simulink model "GMPP2"  (Simulink 8.7)
settings: Solver=ode15s  StartTime=0.0  StopTime=0.3  RelTol=1e-3
libraries: powerlib x29, simulink x13, neural x6
(part 1 of 2)
settings Model: Creator=Loubna  LastModifiedBy=dell
settings DebuggingCC: UnderspecifiedInitializationDetection=Simplified  MergeDetectMultiDrivingBlocksExec=error  SolverPrmCheckMsg=warning
settings ConfigComp: CovSFcnEnable=off

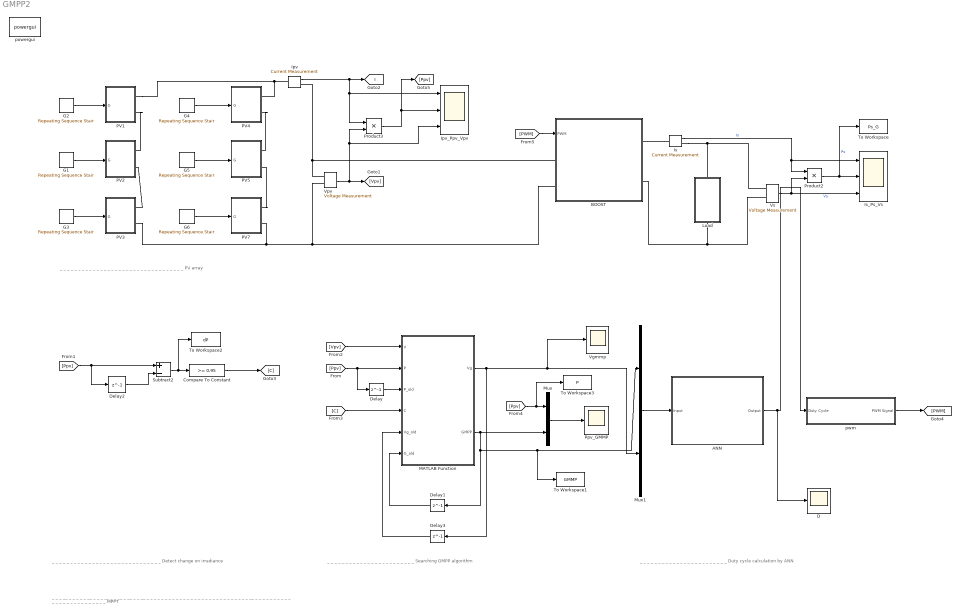
== system GMPP2 ==
  note: _ _ _ _ _ _ _ _ _ _ _ _ _ _ _ _ _ _ _ _ _ _ _ _ _ _ _ _ _ _
      | Detect change on irradiance
  note: _ _ _ _ _ _ _ _ _ _ _ _ _ _ _ _ _ _ _ _ _ _ _ _ _ _ _ _ _ _ _ _ _ _
      | PV array
  note: _ _ _ _ _ _ _ _ _ _ _ _ _ _ _ _ _ _ _ _ _ _ _ _
      | Searching GMPP algorithm
  note: _ _ _ _ _ _ _ _ _ _ _ _ _ _ _ _ _ _ _ _ _ _ _ _
      | Duty cycle calculation by ANN
  note: _ _ _ __ _ _ _ _ _ __ _ _ _ __ _ _ __ _ __ _ _ __ _ _ _ _ _ _ _ _ _ _ _ _ _ _ _ _ _ _ _ _ _ _ _ _ _ _ _ _ __ _ _ _ _ _ _ _ _ _ _ _ _ _ _ _ _ _ _ _ _ _ _ _ _ _
      | MPPT
  ANN : Subsystem
      mask help: Function Fitting Neural Network
      mask Display: e = 0.06;c1 = [120 150 230]/255;c2 = ([120 150 230]+0)/383;c3 = ([120 150 230]+128)/383;patch([0 1 1 0],[0 0 1 1],c1);patch([0 1 1 1-e 1-e 0+e],[0 0 1 1-e 0+e 0+e],c2);patch([0 0 1 1-e 0+e 0+e],[0 1 1 1-e 1-e 0+e],c3);plot([0 1 1 0 0],[0 0 1 1 0]);fprintf('NNET');port_label('input',1,' Input');port_label('output',1,'Output ');
  BOOST : Subsystem
  Compare To Constant : simulink/Logic and Bit Operations/Compare To Constant  relop=>=  const=0.95  OutDataTypeStr=boolean
  D : Scope
  Delay : Delay  DelayLength=1  InitialCondition=0  SampleTime=1e-7
  Delay1 : Delay  DelayLength=1  InitialCondition=0  SampleTime=1e-6
  Delay2 : Delay  DelayLength=1  InitialCondition=0  SampleTime=1e-7
  Delay3 : Delay  DelayLength=1  InitialCondition=0  SampleTime=1e-6
  G1 : simulink/Sources/Repeating Sequence Stair  OutValues=[520 800 560]  tsamp=0.1  OutMin=[]  OutMax=[]  OutDataTypeStr=double  OutputDataTypeScalingMode=double  OutDataType=fixdt(0,8)  ConRadixGroup=Best Precision: Vector-wise  OutScaling=2^-12
  G2 : simulink/Sources/Repeating Sequence Stair  OutValues=[400 550 720]  tsamp=0.1  OutMin=[]  OutMax=[]  OutDataTypeStr=double  OutputDataTypeScalingMode=double  OutDataType=fixdt(0,8)  ConRadixGroup=Best Precision: Vector-wise  OutScaling=2^-12
  G3 : simulink/Sources/Repeating Sequence Stair  OutValues=[700 800 600]  tsamp=0.1  OutMin=[]  OutMax=[]  OutDataTypeStr=double  OutputDataTypeScalingMode=double  OutDataType=fixdt(0,8)  ConRadixGroup=Best Precision: Vector-wise  OutScaling=2^-12
  G4 : simulink/Sources/Repeating Sequence Stair  OutValues=[400 550 560]  tsamp=0.1  OutMin=[]  OutMax=[]  OutDataTypeStr=double  OutputDataTypeScalingMode=double  OutDataType=fixdt(0,8)  ConRadixGroup=Best Precision: Vector-wise  OutScaling=2^-12
  G5 : simulink/Sources/Repeating Sequence Stair  OutValues=[520 800 600]  tsamp=0.1  OutMin=[]  OutMax=[]  OutDataTypeStr=double  OutputDataTypeScalingMode=double  OutDataType=fixdt(0,8)  ConRadixGroup=Best Precision: Vector-wise  OutScaling=2^-12
  G6 : simulink/Sources/Repeating Sequence Stair  OutValues=[700 800 400]  tsamp=0.1  OutMin=[]  OutMax=[]  OutDataTypeStr=double  OutputDataTypeScalingMode=double  OutDataType=fixdt(0,8)  ConRadixGroup=Best Precision: Vector-wise  OutScaling=2^-12
  Ipv : powerlib/Measurements/Current Measurement  PhasorSimulation=off  OutputType=Complex  PSBequivalent=0
  Ipv_Ppv_Vpv : Scope  NumInputPorts=3
  Is : powerlib/Measurements/Current Measurement  PhasorSimulation=off  OutputType=Complex  PSBequivalent=0
  Is_Ps_Vs : Scope  NumInputPorts=3
  Load : Subsystem
  MATLAB Function : MATLAB Function  TreatAsAtomicUnit=on
  Mux : Mux  Inputs=2
  Mux1 : Mux  Inputs=2
  PV1 : Subsystem
  PV2 : Subsystem
  PV3 : Subsystem
  PV4 : Subsystem
  PV5 : Subsystem
  PV7 : Subsystem
  Ppv_GMMP : Scope
  Product2 : Product
  Product3 : Product
  Subtract2 : Sum  Inputs=+-
  To Workspace : ToWorkspace  VariableName=Ps_G  SaveFormat=Timeseries  SampleTime=-1
  To Workspace1 : ToWorkspace  VariableName=GMMP  SaveFormat=Timeseries  SampleTime=-1
  To Workspace2 : ToWorkspace  VariableName=dP  SaveFormat=Timeseries  SampleTime=-1
  To Workspace3 : ToWorkspace  VariableName=P  SaveFormat=Timeseries  SampleTime=-1
  Vgmmp : Scope
  Vpv : powerlib/Measurements/Voltage Measurement  Tag=PoWeRsYsTeMmEaSuReMeNt  PhasorSimulation=off  OutputType=Magnitude  PSBequivalent=0
  Vs : powerlib/Measurements/Voltage Measurement  Tag=PoWeRsYsTeMmEaSuReMeNt  PhasorSimulation=off  OutputType=Magnitude  PSBequivalent=0
  powergui : powerlib/powergui  Priority=1  SimulationMode=Discrete  SolverType=Tustin  SampleTime=1e-6  frequency=60  SPID=off  DisableSnubberDevices=off  DisableRonSwitches=off  DisableVfSwitches=off  SwTol=0  DisplayEquations=off  Interpol=off  ExternalGateDelay=off  methode=off  Ts=0  FunctionMessages=off  echomessages=off  HookPort=off  EnableUseOfTLC=off  x0status=blocks  frequencyindice=0  Pbase=100e6  ErrMax=1e-4  Iterations=50  UnitsV=kV  UnitsW=MW  buscounter=0  RestoreLinks=warning  ResistiveCurrentMeasurement=off  Frange=[0:2:500]  Ylog=off  Xlog=on  ShowGrid=off  save=off  variable=ZData  structure=0  ZoomFFT=off  StartTime=0.0  cycles=1  DisplayStyle=1  fundamental=60  FreqAxis=off  MaxFrequency=1000  frequencyindicesteady=1  RmsSteady=1  display=off
  pwm : Subsystem  mask(PWM Generator for non bridge applications){fs=20000, A=1}
      mask prompts: fs "Frequency"; A "Amplitude"
      mask help:
      | By default it outputs a 1 unit square wave at 1 hz
      | You can set the duty cycle or use an external line to ajust it on the fly.
  tag scope: I=global
  wires:
  Ipv/1 -> Product3/1, Ipv_Ppv_Vpv/1, [I]
  Vpv/1 -> Product3/2, Ipv_Ppv_Vpv/3, [Vpv]
  [Ppv] -> Subtract2/1, Delay2/1
  Delay2/1 -> Subtract2/2
  Subtract2/1 -> To Workspace2/1, Compare To Constant/1
  Delay/1 -> MATLAB Function/3(P_old)
  Delay1/1 -> MATLAB Function/6(G_old)
  Mux/1 -> Ppv_GMMP/1
  [Ppv] -> Delay/1, MATLAB Function/2(P)
  [Vpv] -> MATLAB Function/1(V)
  Mux1/1 -> ANN/1(Input)
  ANN/1(Output) -> pwm/1(Duty Cycle), D/1
  Product2/1 -> To Workspace/1, Is_Ps_Vs/2  "Ps"
  Vs/1 -> Is_Ps_Vs/3, Product2/2  "Vs"
  Is/1 -> Is_Ps_Vs/1, Product2/1  "Is"
  Product3/1 -> [Ppv], Ipv_Ppv_Vpv/2
  Compare To Constant/1 -> [C]
  MATLAB Function/2(GMPP) -> Delay1/1, To Workspace1/1, Mux1/1, Mux/2
  MATLAB Function/1(Vg) -> Delay3/1, Mux1/2, Vgmmp/1
  Delay3/1 -> MATLAB Function/5(Vg_old)
  [Ppv] -> To Workspace3/1, Mux/1
  pwm/1(PWM Signal) -> [PWM]
  [PWM] -> BOOST/1(PWM)
  [C] -> MATLAB Function/4(C)
  G2/1 -> PV1/1(G)
  G3/1 -> PV3/1(G)
  G4/1 -> PV4/1(G)
  G5/1 -> PV5/1(G)
  G6/1 -> PV7/1(G)
  G1/1 -> PV2/1(G)
  connections:
  Vpv/LConn1 -- BOOST/LConn1 -- Ipv/RConn1
  Ipv/LConn1 -- PV4/RConn1 -- PV1/RConn1
  BOOST/LConn2 -- PV3/RConn2 -- PV7/RConn2 -- Vpv/LConn2
  PV1/RConn2 -- PV2/RConn1
  PV4/RConn2 -- PV5/RConn1
  PV7/RConn1 -- PV5/RConn2
  PV3/RConn1 -- PV2/RConn2
  Vs/LConn1 -- Is/RConn1 -- Load/LConn1
  Is/LConn1 -- BOOST/RConn1
  Vs/LConn2 -- BOOST/RConn2 -- Load/RConn1

== system GMPP2/ANN ==
  Input : Inport  PortDimensions=2
      mask Display: e = 0.06;c1 = [120 230 180]/255;c2 = ([120 230 180]+0)/(256+128);c3 = ([120 230 180]+128)/(256+128);patch([0 1 1 0],[0 0 1 1],c1);patch([0 1 1 1-e 1-e 0+e],[0 0 1 1-e 0+e 0+e],c2);patch([0 0 1 1-e 0+e 0+e],[0 1 1 1-e 1-e 0+e],c3);plot([0 1 1 0 0],[0 0 1 1 0]);
  Layer 1 : Subsystem
      mask Display: e = 0.06;c1 = [120 150 230]/255;c2 = ([120 150 230]+0)/383;c3 = ([120 150 230]+128)/383;patch([0 1 1 0],[0 0 1 1],c1);patch([0 1 1 1-e 1-e 0+e],[0 0 1 1-e 0+e 0+e],c2);patch([0 0 1 1-e 0+e 0+e],[0 1 1 1-e 1-e 0+e],c3);plot([0 1 1 0 0],[0 0 1 1 0]);
  Layer 2 : Subsystem
      mask Display: e = 0.06;c1 = [120 150 230]/255;c2 = ([120 150 230]+0)/383;c3 = ([120 150 230]+128)/383;patch([0 1 1 0],[0 0 1 1],c1);patch([0 1 1 1-e 1-e 0+e],[0 0 1 1-e 0+e 0+e],c2);patch([0 0 1 1-e 0+e 0+e],[0 1 1 1-e 1-e 0+e],c3);plot([0 1 1 0 0],[0 0 1 1 0]);
  Process Input 1 : Subsystem
      mask Display: e = 0.06;c1 = [120 150 230]/255;c2 = ([120 150 230]+0)/383;c3 = ([120 150 230]+128)/383;patch([0 1 1 0],[0 0 1 1],c1);patch([0 1 1 1-e 1-e 0+e],[0 0 1 1-e 0+e 0+e],c2);patch([0 0 1 1-e 0+e 0+e],[0 1 1 1-e 1-e 0+e],c3);plot([0 1 1 0 0],[0 0 1 1 0]);
  Process Output 1 : Subsystem
      mask Display: e = 0.06;c1 = [120 150 230]/255;c2 = ([120 150 230]+0)/383;c3 = ([120 150 230]+128)/383;patch([0 1 1 0],[0 0 1 1],c1);patch([0 1 1 1-e 1-e 0+e],[0 0 1 1-e 0+e 0+e],c2);patch([0 0 1 1-e 0+e 0+e],[0 1 1 1-e 1-e 0+e],c3);plot([0 1 1 0 0],[0 0 1 1 0]);
  Output : Outport  InitialOutput=0
      mask Display: e = 0.06;c1 = [120 230 180]/255;c2 = ([120 230 180]+0)/(256+128);c3 = ([120 230 180]+128)/(256+128);patch([0 1 1 0],[0 0 1 1],c1);patch([0 1 1 1-e 1-e 0+e],[0 0 1 1-e 0+e 0+e],c2);patch([0 0 1 1-e 0+e 0+e],[0 1 1 1-e 1-e 0+e],c3);plot([0 1 1 0 0],[0 0 1 1 0]);
  wires:
  Input/1 -> Process Input 1/1(x)
  Process Output 1/1(y) -> Output/1
  Process Input 1/1(p) -> Layer 1/1("p{1}")
  Layer 1/1("a{1}") -> [feedback1]
  [feedback1] -> Layer 2/1("a{1} ")
  Layer 2/1("a{2}") -> Process Output 1/1(a)

== system GMPP2/BOOST ==
  PWM : Inport
  Ce : powerlib/Elements/Series RLC Branch  LConnTagsString=__new0  RConnTagsString=__new0  BranchType=C  Resistance=0.01  Inductance=1.0  SetiL0=off  InitialCurrent=0  Capacitance=10e-6  Setx0=off  InitialVoltage=0  Measurements=None
  Cs : powerlib/Elements/Series RLC Branch  LConnTagsString=__new0  RConnTagsString=__new0  BranchType=C  Resistance=0.01  Inductance=1.0  SetiL0=off  InitialCurrent=0  Capacitance=200e-6  Setx0=off  InitialVoltage=0  Measurements=None
  Diode : powerlib/Power Electronics/Diode  Ron=0.001  Lon=0  Vf=0.8  IC=0  UseSnubber=off  Rs=500  Cs=250e-9  Measurements=off
  Ideal Switch : powerlib/Power Electronics/Ideal Switch  Ron=0.001  Lon=0  IC=0  Rs=1e5  Cs=inf  Measurements=off
  L : powerlib/Elements/Series RLC Branch  LConnTagsString=__new0  RConnTagsString=__new0  BranchType=L  Resistance=0.01  Inductance=10e-3  SetiL0=on  InitialCurrent=0  Capacitance=25e-6  Setx0=off  InitialVoltage=0  Measurements=None
  Vpv+ : PMIOPort  Port=1  Side=Left
  Vs+ : PMIOPort  Port=2  Side=Right
  Vpv- : PMIOPort  Port=3  Side=Left
  Vs- : PMIOPort  Port=4  Side=Right
  wires:
  PWM/1 -> Ideal Switch/1
  connections:
  Diode/LConn1 -- L/LConn1 -- Ideal Switch/LConn1
  Cs/LConn1 -- Vs+/RConn1 -- Diode/RConn1
  Vpv-/RConn1 -- Cs/RConn1 -- Vs-/RConn1 -- Ideal Switch/RConn1 -- Ce/RConn1
  L/RConn1 -- Ce/LConn1 -- Vpv+/RConn1

== system GMPP2/Load ==
  R : powerlib/Elements/Series RLC Branch  LConnTagsString=__new0  RConnTagsString=__new0  BranchType=R  Resistance=15  Inductance=1.0  SetiL0=off  InitialCurrent=0  Capacitance=80e-6  Setx0=off  InitialVoltage=0  Measurements=None
  Vs+ : PMIOPort  Port=1  Side=Left
  Vs- : PMIOPort  Port=2  Side=Right
  connections:
  R/RConn1 -- Vs-/RConn1
  Vs+/RConn1 -- R/LConn1

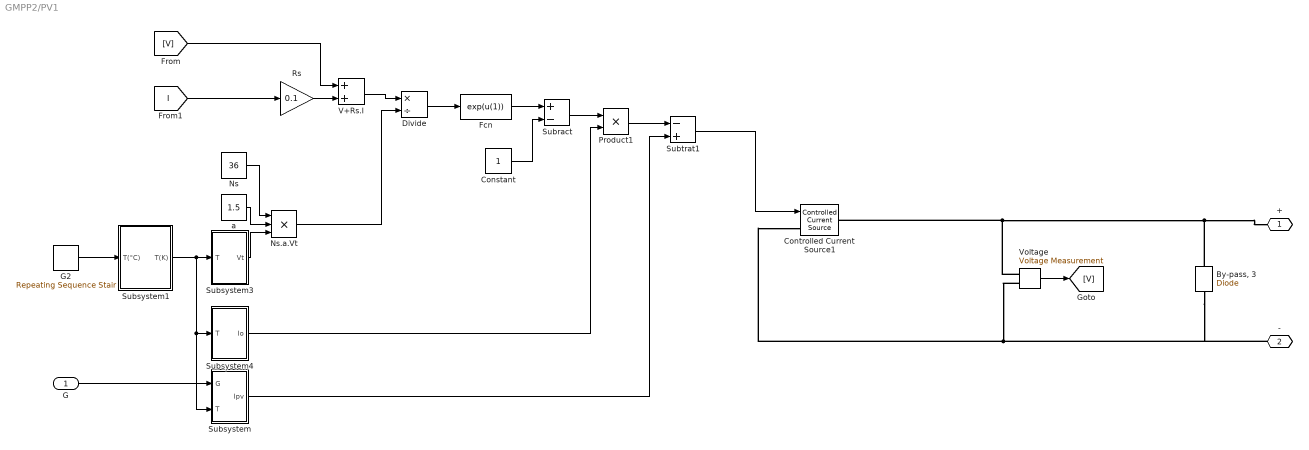
== system GMPP2/PV1 ==
  G : Inport
  "By-pass, 3" : powerlib/Power Electronics/Diode  Ron=0.01  Lon=10e-3  Vf=0.6  IC=0  UseSnubber=off  Rs=0  Cs=250e-9  Measurements=off
  Constant : Constant
  Controlled Current Source1 : powerlib/Electrical Sources/Controlled Current Source  Initialize=on  Source_Type=AC  Amplitude=0  Phase=0  Frequency=0  Measurements=None
  Divide : Product  Inputs=*/
  Fcn : Fcn  Expr=exp(u(1))
  G2 : simulink/Sources/Repeating Sequence Stair  OutValues=[25]  tsamp=0.1  OutMin=[]  OutMax=[]  OutDataTypeStr=double  OutputDataTypeScalingMode=double  OutDataType=fixdt(0,8)  ConRadixGroup=Best Precision: Vector-wise  OutScaling=2^-12
  Ns : Constant  Value=36
  Ns.a.Vt : Product  Inputs=3  RndMeth=Zero
  Product1 : Product  RndMeth=Zero
  Rs : Gain  Gain=0.1
  Subract : Sum  Inputs=+-
  Subsystem : Subsystem
  Subsystem1 : Subsystem
  Subsystem3 : Subsystem
  Subsystem4 : Subsystem
  Subtrat1 : Sum  Inputs=-+
  V+Rs.I : Sum
  "Voltage " : powerlib/Measurements/Voltage Measurement  PhasorSimulation=off  OutputType=Complex  PSBequivalent=0
  a : Constant  Value=1.5
  + : PMIOPort  Port=1  Side=Right
  - : PMIOPort  Port=2  Side=Right
  wires:
  V+Rs.I/1 -> Divide/1
  Divide/1 -> Fcn/1
  Fcn/1 -> Subract/1
  Constant/1 -> Subract/2
  Subract/1 -> Product1/1
  Subsystem4/1(Io) -> Product1/2
  Product1/1 -> Subtrat1/1
  Subsystem1/1(T(K)) -> Subsystem3/1(T), Subsystem4/1(T), Subsystem/2(T)
  G/1 -> Subsystem/1(G)
  Subtrat1/1 -> Controlled Current Source1/1
  G2/1 -> Subsystem1/1(T(°C))
  Ns/1 -> Ns.a.Vt/1
  a/1 -> Ns.a.Vt/2
  Subsystem3/1(Vt) -> Ns.a.Vt/3
  Subsystem/1(Ipv) -> Subtrat1/2
  "Voltage "/1 -> [V]
  Rs/1 -> V+Rs.I/2
  Ns.a.Vt/1 -> Divide/2
  [I] -> Rs/1
  [V] -> V+Rs.I/1
  connections:
  "Voltage "/LConn2 -- -/RConn1 -- "By-pass, 3"/LConn1 -- Controlled Current Source1/LConn1
  "Voltage "/LConn1 -- Controlled Current Source1/RConn1 -- "By-pass, 3"/RConn1 -- +/RConn1

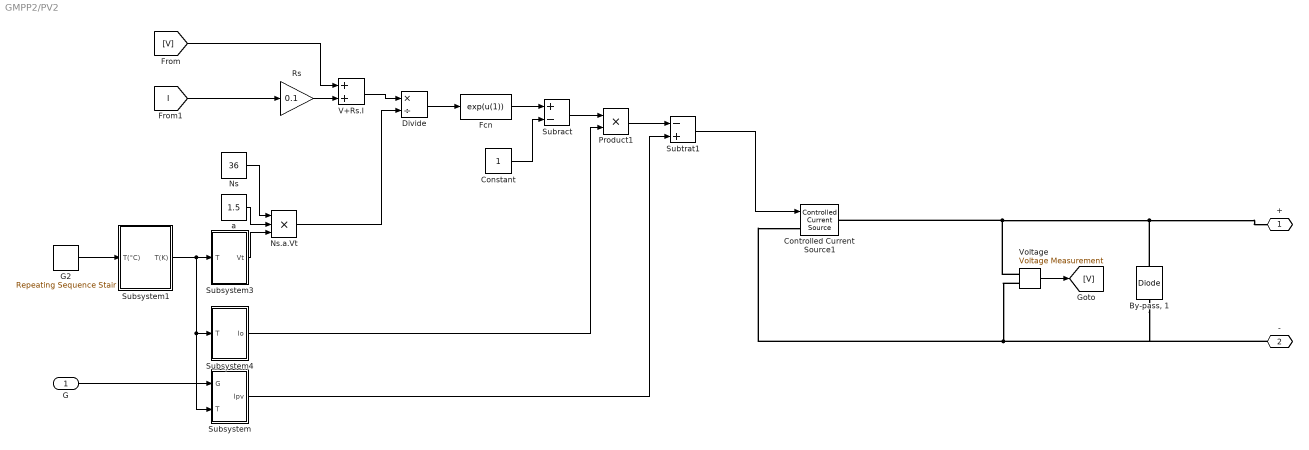
== system GMPP2/PV2 ==
  G : Inport
  "By-pass, 1" : powerlib/Power Electronics/Diode  Ron=0.01  Lon=10e-3  Vf=0.6  IC=0  UseSnubber=off  Rs=0  Cs=250e-9  Measurements=off
  Constant : Constant
  Controlled Current Source1 : powerlib/Electrical Sources/Controlled Current Source  Initialize=on  Source_Type=AC  Amplitude=0  Phase=0  Frequency=0  Measurements=None
  Divide : Product  Inputs=*/
  Fcn : Fcn  Expr=exp(u(1))
  G2 : simulink/Sources/Repeating Sequence Stair  OutValues=[25]  tsamp=0.1  OutMin=[]  OutMax=[]  OutDataTypeStr=double  OutputDataTypeScalingMode=double  OutDataType=fixdt(0,8)  ConRadixGroup=Best Precision: Vector-wise  OutScaling=2^-12
  Ns : Constant  Value=36
  Ns.a.Vt : Product  Inputs=3  RndMeth=Zero
  Product1 : Product  RndMeth=Zero
  Rs : Gain  Gain=0.1
  Subract : Sum  Inputs=+-
  Subsystem : Subsystem
  Subsystem1 : Subsystem
  Subsystem3 : Subsystem
  Subsystem4 : Subsystem
  Subtrat1 : Sum  Inputs=-+
  V+Rs.I : Sum
  "Voltage " : powerlib/Measurements/Voltage Measurement  PhasorSimulation=off  OutputType=Complex  PSBequivalent=0
  a : Constant  Value=1.5
  + : PMIOPort  Port=1  Side=Right
  - : PMIOPort  Port=2  Side=Right
  wires:
  V+Rs.I/1 -> Divide/1
  Divide/1 -> Fcn/1
  Fcn/1 -> Subract/1
  Constant/1 -> Subract/2
  Subract/1 -> Product1/1
  Subsystem4/1(Io) -> Product1/2
  Product1/1 -> Subtrat1/1
  Subsystem1/1(T(K)) -> Subsystem3/1(T), Subsystem4/1(T), Subsystem/2(T)
  G/1 -> Subsystem/1(G)
  Subtrat1/1 -> Controlled Current Source1/1
  G2/1 -> Subsystem1/1(T(°C))
  Ns/1 -> Ns.a.Vt/1
  a/1 -> Ns.a.Vt/2
  Subsystem3/1(Vt) -> Ns.a.Vt/3
  Subsystem/1(Ipv) -> Subtrat1/2
  "Voltage "/1 -> [V]
  Rs/1 -> V+Rs.I/2
  Ns.a.Vt/1 -> Divide/2
  [I] -> Rs/1
  [V] -> V+Rs.I/1
  connections:
  "Voltage "/LConn2 -- "By-pass, 1"/LConn1 -- -/RConn1 -- Controlled Current Source1/LConn1
  "Voltage "/LConn1 -- Controlled Current Source1/RConn1 -- "By-pass, 1"/RConn1 -- +/RConn1

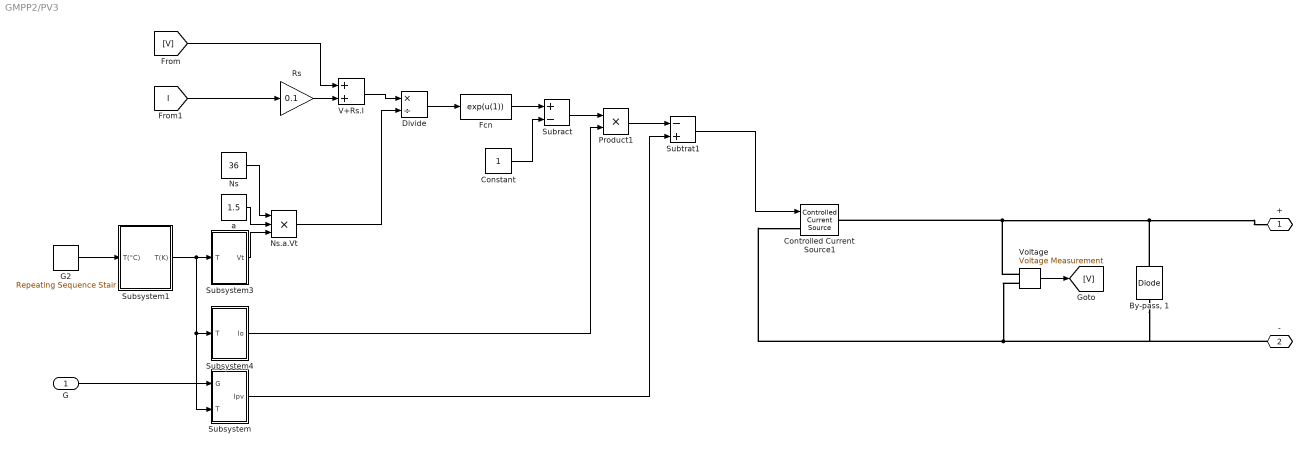
== system GMPP2/PV3 ==
  G : Inport
  "By-pass, 1" : powerlib/Power Electronics/Diode  Ron=0.01  Lon=10e-3  Vf=0.6  IC=0  UseSnubber=off  Rs=0  Cs=250e-9  Measurements=off
  Constant : Constant
  Controlled Current Source1 : powerlib/Electrical Sources/Controlled Current Source  Initialize=on  Source_Type=AC  Amplitude=0  Phase=0  Frequency=0  Measurements=None
  Divide : Product  Inputs=*/
  Fcn : Fcn  Expr=exp(u(1))
  G2 : simulink/Sources/Repeating Sequence Stair  OutValues=[25]  tsamp=0.1  OutMin=[]  OutMax=[]  OutDataTypeStr=double  OutputDataTypeScalingMode=double  OutDataType=fixdt(0,8)  ConRadixGroup=Best Precision: Vector-wise  OutScaling=2^-12
  Ns : Constant  Value=36
  Ns.a.Vt : Product  Inputs=3  RndMeth=Zero
  Product1 : Product  RndMeth=Zero
  Rs : Gain  Gain=0.1
  Subract : Sum  Inputs=+-
  Subsystem : Subsystem
  Subsystem1 : Subsystem
  Subsystem3 : Subsystem
  Subsystem4 : Subsystem
  Subtrat1 : Sum  Inputs=-+
  V+Rs.I : Sum
  "Voltage " : powerlib/Measurements/Voltage Measurement  PhasorSimulation=off  OutputType=Complex  PSBequivalent=0
  a : Constant  Value=1.5
  + : PMIOPort  Port=1  Side=Right
  - : PMIOPort  Port=2  Side=Right
  wires:
  V+Rs.I/1 -> Divide/1
  Divide/1 -> Fcn/1
  Fcn/1 -> Subract/1
  Constant/1 -> Subract/2
  Subract/1 -> Product1/1
  Subsystem4/1(Io) -> Product1/2
  Product1/1 -> Subtrat1/1
  Subsystem1/1(T(K)) -> Subsystem3/1(T), Subsystem4/1(T), Subsystem/2(T)
  G/1 -> Subsystem/1(G)
  Subtrat1/1 -> Controlled Current Source1/1
  G2/1 -> Subsystem1/1(T(°C))
  Ns/1 -> Ns.a.Vt/1
  a/1 -> Ns.a.Vt/2
  Subsystem3/1(Vt) -> Ns.a.Vt/3
  Subsystem/1(Ipv) -> Subtrat1/2
  "Voltage "/1 -> [V]
  Rs/1 -> V+Rs.I/2
  Ns.a.Vt/1 -> Divide/2
  [I] -> Rs/1
  [V] -> V+Rs.I/1
  connections:
  "Voltage "/LConn2 -- "By-pass, 1"/LConn1 -- -/RConn1 -- Controlled Current Source1/LConn1
  "Voltage "/LConn1 -- Controlled Current Source1/RConn1 -- "By-pass, 1"/RConn1 -- +/RConn1

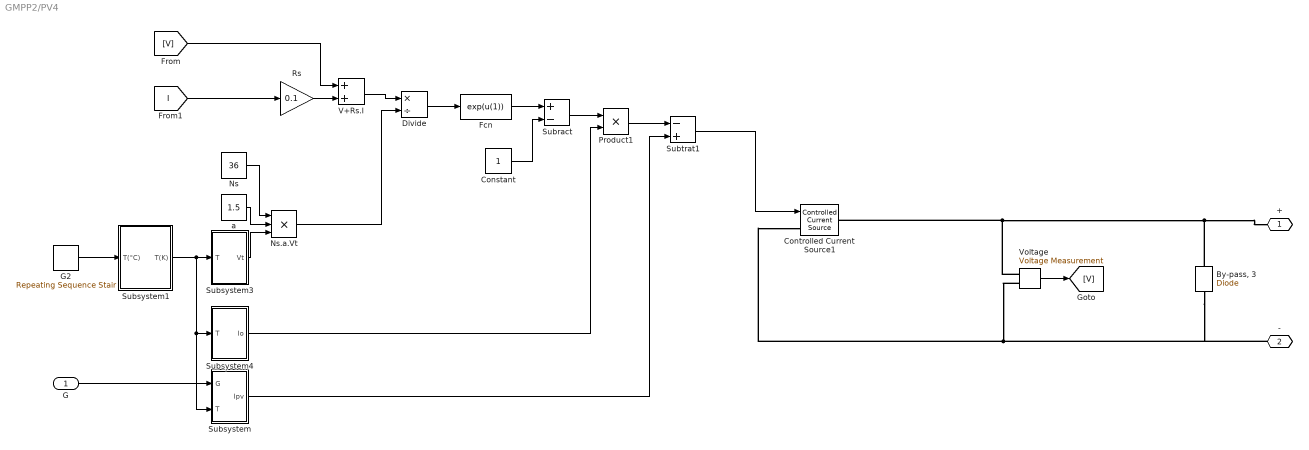
== system GMPP2/PV4 ==
  G : Inport
  "By-pass, 3" : powerlib/Power Electronics/Diode  Ron=0.01  Lon=10e-3  Vf=0.6  IC=0  UseSnubber=off  Rs=0  Cs=250e-9  Measurements=off
  Constant : Constant
  Controlled Current Source1 : powerlib/Electrical Sources/Controlled Current Source  Initialize=on  Source_Type=AC  Amplitude=0  Phase=0  Frequency=0  Measurements=None
  Divide : Product  Inputs=*/
  Fcn : Fcn  Expr=exp(u(1))
  G2 : simulink/Sources/Repeating Sequence Stair  OutValues=[25]  tsamp=0.1  OutMin=[]  OutMax=[]  OutDataTypeStr=double  OutputDataTypeScalingMode=double  OutDataType=fixdt(0,8)  ConRadixGroup=Best Precision: Vector-wise  OutScaling=2^-12
  Ns : Constant  Value=36
  Ns.a.Vt : Product  Inputs=3  RndMeth=Zero
  Product1 : Product  RndMeth=Zero
  Rs : Gain  Gain=0.1
  Subract : Sum  Inputs=+-
  Subsystem : Subsystem
  Subsystem1 : Subsystem
  Subsystem3 : Subsystem
  Subsystem4 : Subsystem
  Subtrat1 : Sum  Inputs=-+
  V+Rs.I : Sum
  "Voltage " : powerlib/Measurements/Voltage Measurement  PhasorSimulation=off  OutputType=Complex  PSBequivalent=0
  a : Constant  Value=1.5
  + : PMIOPort  Port=1  Side=Right
  - : PMIOPort  Port=2  Side=Right
  wires:
  V+Rs.I/1 -> Divide/1
  Divide/1 -> Fcn/1
  Fcn/1 -> Subract/1
  Constant/1 -> Subract/2
  Subract/1 -> Product1/1
  Subsystem4/1(Io) -> Product1/2
  Product1/1 -> Subtrat1/1
  Subsystem1/1(T(K)) -> Subsystem3/1(T), Subsystem4/1(T), Subsystem/2(T)
  G/1 -> Subsystem/1(G)
  Subtrat1/1 -> Controlled Current Source1/1
  G2/1 -> Subsystem1/1(T(°C))
  Ns/1 -> Ns.a.Vt/1
  a/1 -> Ns.a.Vt/2
  Subsystem3/1(Vt) -> Ns.a.Vt/3
  Subsystem/1(Ipv) -> Subtrat1/2
  "Voltage "/1 -> [V]
  Rs/1 -> V+Rs.I/2
  Ns.a.Vt/1 -> Divide/2
  [I] -> Rs/1
  [V] -> V+Rs.I/1
  connections:
  "Voltage "/LConn2 -- -/RConn1 -- "By-pass, 3"/LConn1 -- Controlled Current Source1/LConn1
  "Voltage "/LConn1 -- Controlled Current Source1/RConn1 -- "By-pass, 3"/RConn1 -- +/RConn1

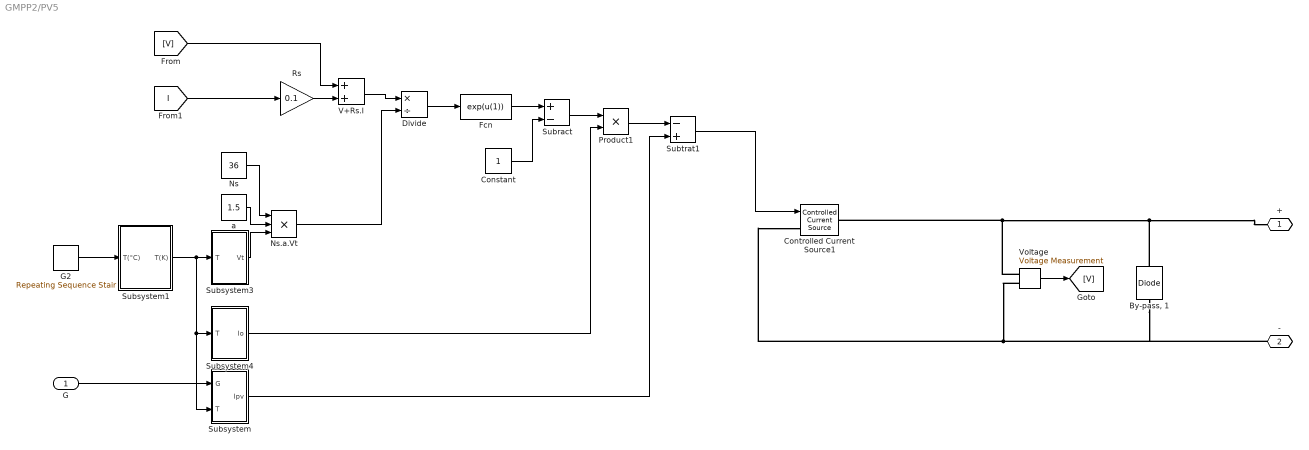
== system GMPP2/PV5 ==
  G : Inport
  "By-pass, 1" : powerlib/Power Electronics/Diode  Ron=0.01  Lon=10e-3  Vf=0.6  IC=0  UseSnubber=off  Rs=0  Cs=250e-9  Measurements=off
  Constant : Constant
  Controlled Current Source1 : powerlib/Electrical Sources/Controlled Current Source  Initialize=on  Source_Type=AC  Amplitude=0  Phase=0  Frequency=0  Measurements=None
  Divide : Product  Inputs=*/
  Fcn : Fcn  Expr=exp(u(1))
  G2 : simulink/Sources/Repeating Sequence Stair  OutValues=[ 25]  tsamp=0.1  OutMin=[]  OutMax=[]  OutDataTypeStr=double  OutputDataTypeScalingMode=double  OutDataType=fixdt(0,8)  ConRadixGroup=Best Precision: Vector-wise  OutScaling=2^-12
  Ns : Constant  Value=36
  Ns.a.Vt : Product  Inputs=3  RndMeth=Zero
  Product1 : Product  RndMeth=Zero
  Rs : Gain  Gain=0.1
  Subract : Sum  Inputs=+-
  Subsystem : Subsystem
  Subsystem1 : Subsystem
  Subsystem3 : Subsystem
  Subsystem4 : Subsystem
  Subtrat1 : Sum  Inputs=-+
  V+Rs.I : Sum
  "Voltage " : powerlib/Measurements/Voltage Measurement  PhasorSimulation=off  OutputType=Complex  PSBequivalent=0
  a : Constant  Value=1.5
  + : PMIOPort  Port=1  Side=Right
  - : PMIOPort  Port=2  Side=Right
  wires:
  V+Rs.I/1 -> Divide/1
  Divide/1 -> Fcn/1
  Fcn/1 -> Subract/1
  Constant/1 -> Subract/2
  Subract/1 -> Product1/1
  Subsystem4/1(Io) -> Product1/2
  Product1/1 -> Subtrat1/1
  Subsystem1/1(T(K)) -> Subsystem3/1(T), Subsystem4/1(T), Subsystem/2(T)
  G/1 -> Subsystem/1(G)
  Subtrat1/1 -> Controlled Current Source1/1
  G2/1 -> Subsystem1/1(T(°C))
  Ns/1 -> Ns.a.Vt/1
  a/1 -> Ns.a.Vt/2
  Subsystem3/1(Vt) -> Ns.a.Vt/3
  Subsystem/1(Ipv) -> Subtrat1/2
  "Voltage "/1 -> [V]
  Rs/1 -> V+Rs.I/2
  Ns.a.Vt/1 -> Divide/2
  [I] -> Rs/1
  [V] -> V+Rs.I/1
  connections:
  "Voltage "/LConn2 -- "By-pass, 1"/LConn1 -- -/RConn1 -- Controlled Current Source1/LConn1
  "Voltage "/LConn1 -- Controlled Current Source1/RConn1 -- "By-pass, 1"/RConn1 -- +/RConn1

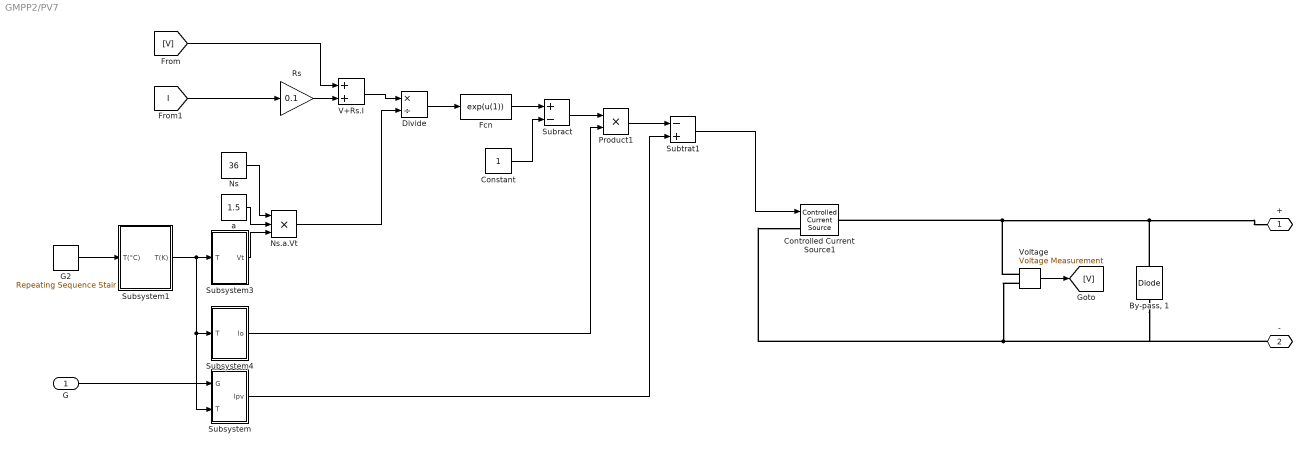
== system GMPP2/PV7 ==
  G : Inport
  "By-pass, 1" : powerlib/Power Electronics/Diode  Ron=0.01  Lon=10e-3  Vf=0.6  IC=0  UseSnubber=off  Rs=0  Cs=250e-9  Measurements=off
  Constant : Constant
  Controlled Current Source1 : powerlib/Electrical Sources/Controlled Current Source  Initialize=on  Source_Type=AC  Amplitude=0  Phase=0  Frequency=0  Measurements=None
  Divide : Product  Inputs=*/
  Fcn : Fcn  Expr=exp(u(1))
  G2 : simulink/Sources/Repeating Sequence Stair  OutValues=[25]  tsamp=0.1  OutMin=[]  OutMax=[]  OutDataTypeStr=double  OutputDataTypeScalingMode=double  OutDataType=fixdt(0,8)  ConRadixGroup=Best Precision: Vector-wise  OutScaling=2^-12
  Ns : Constant  Value=36
  Ns.a.Vt : Product  Inputs=3  RndMeth=Zero
  Product1 : Product  RndMeth=Zero
  Rs : Gain  Gain=0.1
  Subract : Sum  Inputs=+-
  Subsystem : Subsystem
  Subsystem1 : Subsystem
  Subsystem3 : Subsystem
  Subsystem4 : Subsystem
  Subtrat1 : Sum  Inputs=-+
  V+Rs.I : Sum
  "Voltage " : powerlib/Measurements/Voltage Measurement  PhasorSimulation=off  OutputType=Complex  PSBequivalent=0
  a : Constant  Value=1.5
  + : PMIOPort  Port=1  Side=Right
  - : PMIOPort  Port=2  Side=Right
  wires:
  V+Rs.I/1 -> Divide/1
  Divide/1 -> Fcn/1
  Fcn/1 -> Subract/1
  Constant/1 -> Subract/2
  Subract/1 -> Product1/1
  Subsystem4/1(Io) -> Product1/2
  Product1/1 -> Subtrat1/1
  Subsystem1/1(T(K)) -> Subsystem3/1(T), Subsystem4/1(T), Subsystem/2(T)
  G/1 -> Subsystem/1(G)
  Subtrat1/1 -> Controlled Current Source1/1
  G2/1 -> Subsystem1/1(T(°C))
  Ns/1 -> Ns.a.Vt/1
  a/1 -> Ns.a.Vt/2
  Subsystem3/1(Vt) -> Ns.a.Vt/3
  Subsystem/1(Ipv) -> Subtrat1/2
  "Voltage "/1 -> [V]
  Rs/1 -> V+Rs.I/2
  Ns.a.Vt/1 -> Divide/2
  [I] -> Rs/1
  [V] -> V+Rs.I/1
  connections:
  "Voltage "/LConn2 -- "By-pass, 1"/LConn1 -- -/RConn1 -- Controlled Current Source1/LConn1
  "Voltage "/LConn1 -- Controlled Current Source1/RConn1 -- "By-pass, 1"/RConn1 -- +/RConn1

== system GMPP2/pwm ==
  note: Duty Cycle 0.01 < D < 0.99
  Duty Cycle : Inport
  Gain : Gain  Gain=A
  Saturation : Saturate  UpperLimit=1  LowerLimit=0
  Saturation1 : Saturate  UpperLimit=0.99  LowerLimit=0.01
  Sign : Signum
  Sum : Sum  Inputs=|-+
  saw wave : Subsystem  mask{fs=fs}
      mask init:
      | x=[-1 NaN 4 NaN 0 1 1 2 2 3 3];
      | y=[-0.5 NaN 1.5 NaN 0 1 0 1 0 1 0];
      mask Display:
      | plot(x,y);
      | port_label('output',1,'S')
  PWM Signal : Outport
  wires:
  saw wave/1(Out1) -> Sum/1
  Sum/1 -> Sign/1
  Sign/1 -> Saturation/1
  Saturation/1 -> Gain/1
  Gain/1 -> PWM Signal/1
  Saturation1/1 -> Sum/2
  Duty Cycle/1 -> Saturation1/1

== system GMPP2/ANN/Layer 1 ==
  "p{1}" : Inport  PortDimensions=2
      mask Display: e = 0.06;c1 = [120 230 180]/255;c2 = ([120 230 180]+0)/(256+128);c3 = ([120 230 180]+128)/(256+128);patch([0 1 1 0],[0 0 1 1],c1);patch([0 1 1 1-e 1-e 0+e],[0 0 1 1-e 0+e 0+e],c2);patch([0 0 1 1-e 0+e 0+e],[0 1 1 1-e 1-e 0+e],c3);plot([0 1 1 0 0],[0 0 1 1 0]);
  Delays 1 : Subsystem
      mask Display: e = 0.06;c1 = [120 150 230]/255;c2 = ([120 150 230]+0)/383;c3 = ([120 150 230]+128)/383;patch([0 1 1 0],[0 0 1 1],c1);patch([0 1 1 1-e 1-e 0+e],[0 0 1 1-e 0+e 0+e],c2);patch([0 0 1 1-e 0+e 0+e],[0 1 1 1-e 1-e 0+e],c3);plot([0 1 1 0 0],[0 0 1 1 0]);disp('0');
  "IW{1,1}" : Subsystem
      mask Display: e = 0.06;c1 = [120 150 230]/255;c2 = ([120 150 230]+0)/383;c3 = ([120 150 230]+128)/383;patch([0 1 1 0],[0 0 1 1],c1);patch([0 1 1 1-e 1-e 0+e],[0 0 1 1-e 0+e 0+e],c2);patch([0 0 1 1-e 0+e 0+e],[0 1 1 1-e 1-e 0+e],c3);plot([0 1 1 0 0],[0 0 1 1 0]);disp('W');
  "b{1}" : Constant  Value=2.1105511112631157
      mask Display: e = 0.06;c1 = [120 150 230]/255;c2 = ([120 150 230]+0)/383;c3 = ([120 150 230]+128)/383;patch([0 1 1 0],[0 0 1 1],c1);patch([0 1 1 1-e 1-e 0+e],[0 0 1 1-e 0+e 0+e],c2);patch([0 0 1 1-e 0+e 0+e],[0 1 1 1-e 1-e 0+e],c3);plot([0 1 1 0 0],[0 0 1 1 0]);disp('b');
  netsum : Sum  Inputs=2  SaturateOnIntegerOverflow=on  InputSameDT=on  OutDataTypeStr=Inherit: Same as first input
      mask Display: e = 0.06;c1 = [120 150 230]/255;c2 = ([120 150 230]+0)/383;c3 = ([120 150 230]+128)/383;patch([0 1 1 0],[0 0 1 1],c1);patch([0 1 1 1-e 1-e 0+e],[0 0 1 1-e 0+e 0+e],c2);patch([0 0 1 1-e 0+e 0+e],[0 1 1 1-e 1-e 0+e],c3);plot([0 1 1 0 0],[0 0 1 1 0]);disp('+');
  tansig : neural/Transfer Functions/tansig
  "a{1}" : Outport  InitialOutput=0
      mask Display: e = 0.06;c1 = [120 230 180]/255;c2 = ([120 230 180]+0)/(256+128);c3 = ([120 230 180]+128)/(256+128);patch([0 1 1 0],[0 0 1 1],c1);patch([0 1 1 1-e 1-e 0+e],[0 0 1 1-e 0+e 0+e],c2);patch([0 0 1 1-e 0+e 0+e],[0 1 1 1-e 1-e 0+e],c3);plot([0 1 1 0 0],[0 0 1 1 0]);
  wires:
  "p{1}"/1 -> Delays 1/1("p{1}")
  Delays 1/1("pd{1,1}") -> "IW{1,1}"/1("pd{1,1}")
  "IW{1,1}"/1("iz{1,1}") -> netsum/1
  "b{1}"/1 -> netsum/2
  netsum/1 -> tansig/1
  tansig/1 -> "a{1}"/1

== system GMPP2/ANN/Layer 2 ==
  "a{1} " : Inport  PortDimensions=1
      mask Display: e = 0.06;c1 = [120 230 180]/255;c2 = ([120 230 180]+0)/(256+128);c3 = ([120 230 180]+128)/(256+128);patch([0 1 1 0],[0 0 1 1],c1);patch([0 1 1 1-e 1-e 0+e],[0 0 1 1-e 0+e 0+e],c2);patch([0 0 1 1-e 0+e 0+e],[0 1 1 1-e 1-e 0+e],c3);plot([0 1 1 0 0],[0 0 1 1 0]);
  Delays 1 : Subsystem
      mask Display: e = 0.06;c1 = [120 150 230]/255;c2 = ([120 150 230]+0)/383;c3 = ([120 150 230]+128)/383;patch([0 1 1 0],[0 0 1 1],c1);patch([0 1 1 1-e 1-e 0+e],[0 0 1 1-e 0+e 0+e],c2);patch([0 0 1 1-e 0+e 0+e],[0 1 1 1-e 1-e 0+e],c3);plot([0 1 1 0 0],[0 0 1 1 0]);disp('0');
  "LW{2,1}" : Subsystem
      mask Display: e = 0.06;c1 = [120 150 230]/255;c2 = ([120 150 230]+0)/383;c3 = ([120 150 230]+128)/383;patch([0 1 1 0],[0 0 1 1],c1);patch([0 1 1 1-e 1-e 0+e],[0 0 1 1-e 0+e 0+e],c2);patch([0 0 1 1-e 0+e 0+e],[0 1 1 1-e 1-e 0+e],c3);plot([0 1 1 0 0],[0 0 1 1 0]);disp('W');
  "b{2}" : Constant  Value=-23.727405683814752
      mask Display: e = 0.06;c1 = [120 150 230]/255;c2 = ([120 150 230]+0)/383;c3 = ([120 150 230]+128)/383;patch([0 1 1 0],[0 0 1 1],c1);patch([0 1 1 1-e 1-e 0+e],[0 0 1 1-e 0+e 0+e],c2);patch([0 0 1 1-e 0+e 0+e],[0 1 1 1-e 1-e 0+e],c3);plot([0 1 1 0 0],[0 0 1 1 0]);disp('b');
  netsum : Sum  Inputs=2  SaturateOnIntegerOverflow=on  InputSameDT=on  OutDataTypeStr=Inherit: Same as first input
      mask Display: e = 0.06;c1 = [120 150 230]/255;c2 = ([120 150 230]+0)/383;c3 = ([120 150 230]+128)/383;patch([0 1 1 0],[0 0 1 1],c1);patch([0 1 1 1-e 1-e 0+e],[0 0 1 1-e 0+e 0+e],c2);patch([0 0 1 1-e 0+e 0+e],[0 1 1 1-e 1-e 0+e],c3);plot([0 1 1 0 0],[0 0 1 1 0]);disp('+');
  purelin : neural/Transfer Functions/purelin
  "a{2}" : Outport  InitialOutput=0
      mask Display: e = 0.06;c1 = [120 230 180]/255;c2 = ([120 230 180]+0)/(256+128);c3 = ([120 230 180]+128)/(256+128);patch([0 1 1 0],[0 0 1 1],c1);patch([0 1 1 1-e 1-e 0+e],[0 0 1 1-e 0+e 0+e],c2);patch([0 0 1 1-e 0+e 0+e],[0 1 1 1-e 1-e 0+e],c3);plot([0 1 1 0 0],[0 0 1 1 0]);
  wires:
  "a{1} "/1 -> Delays 1/1("p{2}")
  Delays 1/1("pd{2,1}") -> "LW{2,1}"/1("ad{2,1}")
  "LW{2,1}"/1("lz{2,1}") -> netsum/1
  "b{2}"/1 -> netsum/2
  netsum/1 -> purelin/1
  purelin/1 -> "a{2}"/1

== system GMPP2/ANN/Process Input 1 ==
  x : Inport  PortDimensions=2
      mask Display: e = 0.06;c1 = [120 230 180]/255;c2 = ([120 230 180]+0)/(256+128);c3 = ([120 230 180]+128)/(256+128);patch([0 1 1 0],[0 0 1 1],c1);patch([0 1 1 1-e 1-e 0+e],[0 0 1 1-e 0+e 0+e],c2);patch([0 0 1 1-e 0+e 0+e],[0 1 1 1-e 1-e 0+e],c3);plot([0 1 1 0 0],[0 0 1 1 0]);
  mapminmax : neural/Processing Functions/mapminmax  xmin=[149.69;45.189999999999998]  xmax=[675.55999999999995;52.340000000000003]  ymin=-1  ymax=1
  p : Outport  PortDimensions=2
      mask Display: e = 0.06;c1 = [120 230 180]/255;c2 = ([120 230 180]+0)/(256+128);c3 = ([120 230 180]+128)/(256+128);patch([0 1 1 0],[0 0 1 1],c1);patch([0 1 1 1-e 1-e 0+e],[0 0 1 1-e 0+e 0+e],c2);patch([0 0 1 1-e 0+e 0+e],[0 1 1 1-e 1-e 0+e],c3);plot([0 1 1 0 0],[0 0 1 1 0]);
  wires:
  x/1 -> mapminmax/1
  mapminmax/1 -> p/1

== system GMPP2/ANN/Process Output 1 ==
  a : Inport  PortDimensions=1
      mask Display: e = 0.06;c1 = [120 230 180]/255;c2 = ([120 230 180]+0)/(256+128);c3 = ([120 230 180]+128)/(256+128);patch([0 1 1 0],[0 0 1 1],c1);patch([0 1 1 1-e 1-e 0+e],[0 0 1 1-e 0+e 0+e],c2);patch([0 0 1 1-e 0+e 0+e],[0 1 1 1-e 1-e 0+e],c3);plot([0 1 1 0 0],[0 0 1 1 0]);
  mapminmax_reverse : neural/Processing Functions/mapminmax_reverse  xmin=0.045999999999999999  xmax=0.497  ymin=-1  ymax=1
  y : Outport  PortDimensions=1
      mask Display: e = 0.06;c1 = [120 230 180]/255;c2 = ([120 230 180]+0)/(256+128);c3 = ([120 230 180]+128)/(256+128);patch([0 1 1 0],[0 0 1 1],c1);patch([0 1 1 1-e 1-e 0+e],[0 0 1 1-e 0+e 0+e],c2);patch([0 0 1 1-e 0+e 0+e],[0 1 1 1-e 1-e 0+e],c3);plot([0 1 1 0 0],[0 0 1 1 0]);
  wires:
  a/1 -> mapminmax_reverse/1
  mapminmax_reverse/1 -> y/1

== system GMPP2/PV1/Subsystem ==
  G : Inport
  T : Inport  Port=2
  G/Gn : Product  Inputs=*/
  Gn : Constant  Value=1000
  Ipv,n : Constant  Value=7.24
  Ki : Constant  Value=3.18e-3
  Ki.dT : Product  RndMeth=Zero
  Ki.dT+ Ipv,n : Sum
  Product : Product  RndMeth=Zero
  Subsystem2 : Subsystem
  Ipv : Outport
  wires:
  Ki/1 -> Ki.dT/1
  Ipv,n/1 -> Ki.dT+ Ipv,n/1
  Ki.dT/1 -> Ki.dT+ Ipv,n/2
  G/1 -> G/Gn/1
  Gn/1 -> G/Gn/2
  G/Gn/1 -> Product/1
  Ki.dT+ Ipv,n/1 -> Product/2
  Product/1 -> Ipv/1
  Subsystem2/1(dT) -> Ki.dT/2
  T/1 -> Subsystem2/1(T)

== system GMPP2/PV1/Subsystem1 ==
  T(°C) : Inport
  Constant1 : Constant  Value=273.15
  V+Rs.I1 : Sum
  T(K) : Outport
  wires:
  Constant1/1 -> V+Rs.I1/2
  T(°C)/1 -> V+Rs.I1/1
  V+Rs.I1/1 -> T(K)/1

== system GMPP2/PV1/Subsystem3 ==
  T : Inport
  Divide : Product  Inputs=**/
  K : Constant  Value=1.38e-23
  q : Constant  Value=1.6e-19
  Vt : Outport
  wires:
  K/1 -> Divide/1
  T/1 -> Divide/2
  q/1 -> Divide/3
  Divide/1 -> Vt/1

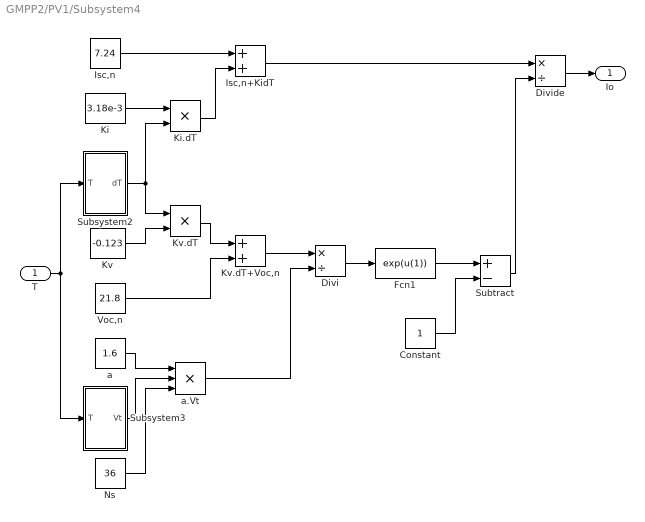
== system GMPP2/PV1/Subsystem4 ==
  T : Inport
  Constant : Constant
  Divi : Product  Inputs=*/
  Divide : Product  Inputs=*/
  Fcn1 : Fcn  Expr=exp(u(1))
  Isc,n : Constant  Value=7.24
  Isc,n+KidT : Sum
  Ki : Constant  Value=3.18e-3
  Ki.dT : Product  RndMeth=Zero
  Kv : Constant  Value=-0.123
  Kv.dT : Product  RndMeth=Zero
  Kv.dT+Voc,n : Sum
  Ns : Constant  Value=36
  Subsystem2 : Subsystem
  Subsystem3 : Subsystem
  Subtract : Sum  Inputs=+-
  Voc,n : Constant  Value=21.8
  a : Constant  Value=1.6
  a.Vt : Product  Inputs=3  RndMeth=Zero
  Io : Outport
  wires:
  Subsystem2/1(dT) -> Kv.dT/1, Ki.dT/2
  Kv/1 -> Kv.dT/2
  Kv.dT/1 -> Kv.dT+Voc,n/1
  Voc,n/1 -> Kv.dT+Voc,n/2
  a/1 -> a.Vt/1
  Subsystem3/1(Vt) -> a.Vt/2
  Kv.dT+Voc,n/1 -> Divi/1
  a.Vt/1 -> Divi/2
  Divi/1 -> Fcn1/1
  Fcn1/1 -> Subtract/1
  Constant/1 -> Subtract/2
  Ki/1 -> Ki.dT/1
  Isc,n/1 -> Isc,n+KidT/1
  Ki.dT/1 -> Isc,n+KidT/2
  Isc,n+KidT/1 -> Divide/1
  Subtract/1 -> Divide/2
  Divide/1 -> Io/1
  T/1 -> Subsystem2/1(T), Subsystem3/1(T)
  Ns/1 -> a.Vt/3

== system GMPP2/PV2/Subsystem ==
  G : Inport
  T : Inport  Port=2
  G/Gn : Product  Inputs=*/
  Gn : Constant  Value=1000
  Ipv,n : Constant  Value=7.24
  Ki : Constant  Value=3.18e-3
  Ki.dT : Product  RndMeth=Zero
  Ki.dT+ Ipv,n : Sum
  Product : Product  RndMeth=Zero
  Subsystem2 : Subsystem
  Ipv : Outport
  wires:
  Ki/1 -> Ki.dT/1
  Ipv,n/1 -> Ki.dT+ Ipv,n/1
  Ki.dT/1 -> Ki.dT+ Ipv,n/2
  G/1 -> G/Gn/1
  Gn/1 -> G/Gn/2
  G/Gn/1 -> Product/1
  Ki.dT+ Ipv,n/1 -> Product/2
  Product/1 -> Ipv/1
  Subsystem2/1(dT) -> Ki.dT/2
  T/1 -> Subsystem2/1(T)

== system GMPP2/PV2/Subsystem1 ==
  T(°C) : Inport
  Constant1 : Constant  Value=273.15
  V+Rs.I1 : Sum
  T(K) : Outport
  wires:
  Constant1/1 -> V+Rs.I1/2
  T(°C)/1 -> V+Rs.I1/1
  V+Rs.I1/1 -> T(K)/1

== system GMPP2/PV2/Subsystem3 ==
  T : Inport
  Divide : Product  Inputs=**/
  K : Constant  Value=1.38e-23
  q : Constant  Value=1.6e-19
  Vt : Outport
  wires:
  K/1 -> Divide/1
  T/1 -> Divide/2
  q/1 -> Divide/3
  Divide/1 -> Vt/1

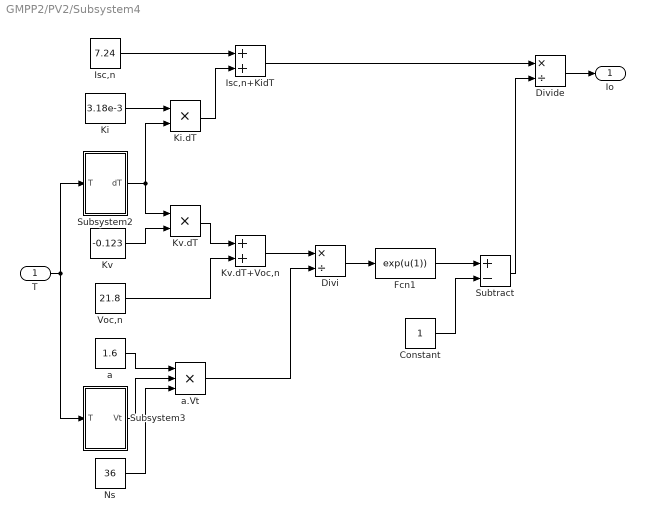
== system GMPP2/PV2/Subsystem4 ==
  T : Inport
  Constant : Constant
  Divi : Product  Inputs=*/
  Divide : Product  Inputs=*/
  Fcn1 : Fcn  Expr=exp(u(1))
  Isc,n : Constant  Value=7.24
  Isc,n+KidT : Sum
  Ki : Constant  Value=3.18e-3
  Ki.dT : Product  RndMeth=Zero
  Kv : Constant  Value=-0.123
  Kv.dT : Product  RndMeth=Zero
  Kv.dT+Voc,n : Sum
  Ns : Constant  Value=36
  Subsystem2 : Subsystem
  Subsystem3 : Subsystem
  Subtract : Sum  Inputs=+-
  Voc,n : Constant  Value=21.8
  a : Constant  Value=1.6
  a.Vt : Product  Inputs=3  RndMeth=Zero
  Io : Outport
  wires:
  Subsystem2/1(dT) -> Kv.dT/1, Ki.dT/2
  Kv/1 -> Kv.dT/2
  Kv.dT/1 -> Kv.dT+Voc,n/1
  Voc,n/1 -> Kv.dT+Voc,n/2
  a/1 -> a.Vt/1
  Subsystem3/1(Vt) -> a.Vt/2
  Kv.dT+Voc,n/1 -> Divi/1
  a.Vt/1 -> Divi/2
  Divi/1 -> Fcn1/1
  Fcn1/1 -> Subtract/1
  Constant/1 -> Subtract/2
  Ki/1 -> Ki.dT/1
  Isc,n/1 -> Isc,n+KidT/1
  Ki.dT/1 -> Isc,n+KidT/2
  Isc,n+KidT/1 -> Divide/1
  Subtract/1 -> Divide/2
  Divide/1 -> Io/1
  T/1 -> Subsystem2/1(T), Subsystem3/1(T)
  Ns/1 -> a.Vt/3

== system GMPP2/PV3/Subsystem ==
  G : Inport
  T : Inport  Port=2
  G/Gn : Product  Inputs=*/
  Gn : Constant  Value=1000
  Ipv,n : Constant  Value=7.24
  Ki : Constant  Value=3.18e-3
  Ki.dT : Product  RndMeth=Zero
  Ki.dT+ Ipv,n : Sum
  Product : Product  RndMeth=Zero
  Subsystem2 : Subsystem
  Ipv : Outport
  wires:
  Ki/1 -> Ki.dT/1
  Ipv,n/1 -> Ki.dT+ Ipv,n/1
  Ki.dT/1 -> Ki.dT+ Ipv,n/2
  G/1 -> G/Gn/1
  Gn/1 -> G/Gn/2
  G/Gn/1 -> Product/1
  Ki.dT+ Ipv,n/1 -> Product/2
  Product/1 -> Ipv/1
  Subsystem2/1(dT) -> Ki.dT/2
  T/1 -> Subsystem2/1(T)

== system GMPP2/PV3/Subsystem1 ==
  T(°C) : Inport
  Constant1 : Constant  Value=273.15
  V+Rs.I1 : Sum
  T(K) : Outport
  wires:
  Constant1/1 -> V+Rs.I1/2
  T(°C)/1 -> V+Rs.I1/1
  V+Rs.I1/1 -> T(K)/1

== system GMPP2/PV3/Subsystem3 ==
  T : Inport
  Divide : Product  Inputs=**/
  K : Constant  Value=1.38e-23
  q : Constant  Value=1.6e-19
  Vt : Outport
  wires:
  K/1 -> Divide/1
  T/1 -> Divide/2
  q/1 -> Divide/3
  Divide/1 -> Vt/1

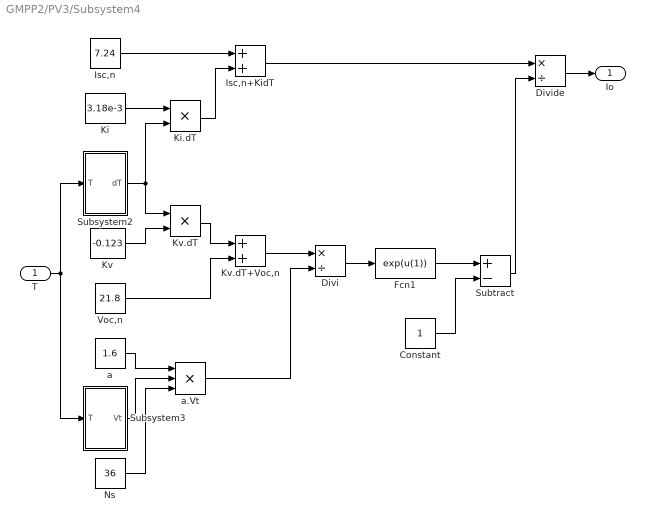
== system GMPP2/PV3/Subsystem4 ==
  T : Inport
  Constant : Constant
  Divi : Product  Inputs=*/
  Divide : Product  Inputs=*/
  Fcn1 : Fcn  Expr=exp(u(1))
  Isc,n : Constant  Value=7.24
  Isc,n+KidT : Sum
  Ki : Constant  Value=3.18e-3
  Ki.dT : Product  RndMeth=Zero
  Kv : Constant  Value=-0.123
  Kv.dT : Product  RndMeth=Zero
  Kv.dT+Voc,n : Sum
  Ns : Constant  Value=36
  Subsystem2 : Subsystem
  Subsystem3 : Subsystem
  Subtract : Sum  Inputs=+-
  Voc,n : Constant  Value=21.8
  a : Constant  Value=1.6
  a.Vt : Product  Inputs=3  RndMeth=Zero
  Io : Outport
  wires:
  Subsystem2/1(dT) -> Kv.dT/1, Ki.dT/2
  Kv/1 -> Kv.dT/2
  Kv.dT/1 -> Kv.dT+Voc,n/1
  Voc,n/1 -> Kv.dT+Voc,n/2
  a/1 -> a.Vt/1
  Subsystem3/1(Vt) -> a.Vt/2
  Kv.dT+Voc,n/1 -> Divi/1
  a.Vt/1 -> Divi/2
  Divi/1 -> Fcn1/1
  Fcn1/1 -> Subtract/1
  Constant/1 -> Subtract/2
  Ki/1 -> Ki.dT/1
  Isc,n/1 -> Isc,n+KidT/1
  Ki.dT/1 -> Isc,n+KidT/2
  Isc,n+KidT/1 -> Divide/1
  Subtract/1 -> Divide/2
  Divide/1 -> Io/1
  T/1 -> Subsystem2/1(T), Subsystem3/1(T)
  Ns/1 -> a.Vt/3

== system GMPP2/PV4/Subsystem ==
  G : Inport
  T : Inport  Port=2
  G/Gn : Product  Inputs=*/
  Gn : Constant  Value=1000
  Ipv,n : Constant  Value=7.24
  Ki : Constant  Value=3.18e-3
  Ki.dT : Product  RndMeth=Zero
  Ki.dT+ Ipv,n : Sum
  Product : Product  RndMeth=Zero
  Subsystem2 : Subsystem
  Ipv : Outport
  wires:
  Ki/1 -> Ki.dT/1
  Ipv,n/1 -> Ki.dT+ Ipv,n/1
  Ki.dT/1 -> Ki.dT+ Ipv,n/2
  G/1 -> G/Gn/1
  Gn/1 -> G/Gn/2
  G/Gn/1 -> Product/1
  Ki.dT+ Ipv,n/1 -> Product/2
  Product/1 -> Ipv/1
  Subsystem2/1(dT) -> Ki.dT/2
  T/1 -> Subsystem2/1(T)

== system GMPP2/PV4/Subsystem1 ==
  T(°C) : Inport
  Constant1 : Constant  Value=273.15
  V+Rs.I1 : Sum
  T(K) : Outport
  wires:
  Constant1/1 -> V+Rs.I1/2
  T(°C)/1 -> V+Rs.I1/1
  V+Rs.I1/1 -> T(K)/1

== system GMPP2/PV4/Subsystem3 ==
  T : Inport
  Divide : Product  Inputs=**/
  K : Constant  Value=1.38e-23
  q : Constant  Value=1.6e-19
  Vt : Outport
  wires:
  K/1 -> Divide/1
  T/1 -> Divide/2
  q/1 -> Divide/3
  Divide/1 -> Vt/1

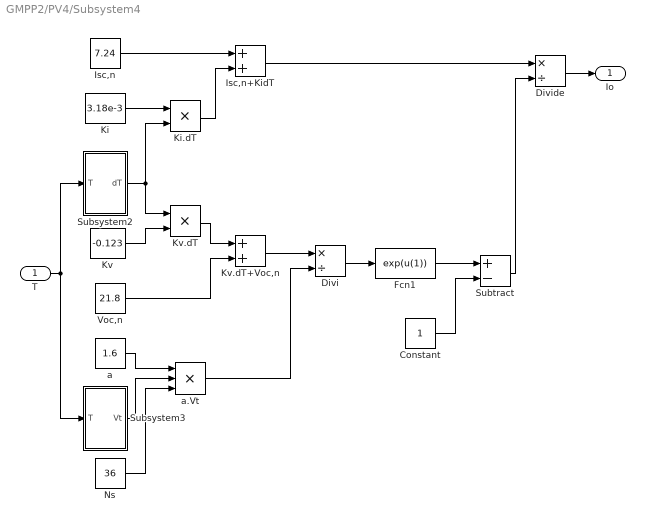
== system GMPP2/PV4/Subsystem4 ==
  T : Inport
  Constant : Constant
  Divi : Product  Inputs=*/
  Divide : Product  Inputs=*/
  Fcn1 : Fcn  Expr=exp(u(1))
  Isc,n : Constant  Value=7.24
  Isc,n+KidT : Sum
  Ki : Constant  Value=3.18e-3
  Ki.dT : Product  RndMeth=Zero
  Kv : Constant  Value=-0.123
  Kv.dT : Product  RndMeth=Zero
  Kv.dT+Voc,n : Sum
  Ns : Constant  Value=36
  Subsystem2 : Subsystem
  Subsystem3 : Subsystem
  Subtract : Sum  Inputs=+-
  Voc,n : Constant  Value=21.8
  a : Constant  Value=1.6
  a.Vt : Product  Inputs=3  RndMeth=Zero
  Io : Outport
  wires:
  Subsystem2/1(dT) -> Kv.dT/1, Ki.dT/2
  Kv/1 -> Kv.dT/2
  Kv.dT/1 -> Kv.dT+Voc,n/1
  Voc,n/1 -> Kv.dT+Voc,n/2
  a/1 -> a.Vt/1
  Subsystem3/1(Vt) -> a.Vt/2
  Kv.dT+Voc,n/1 -> Divi/1
  a.Vt/1 -> Divi/2
  Divi/1 -> Fcn1/1
  Fcn1/1 -> Subtract/1
  Constant/1 -> Subtract/2
  Ki/1 -> Ki.dT/1
  Isc,n/1 -> Isc,n+KidT/1
  Ki.dT/1 -> Isc,n+KidT/2
  Isc,n+KidT/1 -> Divide/1
  Subtract/1 -> Divide/2
  Divide/1 -> Io/1
  T/1 -> Subsystem2/1(T), Subsystem3/1(T)
  Ns/1 -> a.Vt/3

== system GMPP2/PV5/Subsystem ==
  G : Inport
  T : Inport  Port=2
  G/Gn : Product  Inputs=*/
  Gn : Constant  Value=1000
  Ipv,n : Constant  Value=7.24
  Ki : Constant  Value=3.18e-3
  Ki.dT : Product  RndMeth=Zero
  Ki.dT+ Ipv,n : Sum
  Product : Product  RndMeth=Zero
  Subsystem2 : Subsystem
  Ipv : Outport
  wires:
  Ki/1 -> Ki.dT/1
  Ipv,n/1 -> Ki.dT+ Ipv,n/1
  Ki.dT/1 -> Ki.dT+ Ipv,n/2
  G/1 -> G/Gn/1
  Gn/1 -> G/Gn/2
  G/Gn/1 -> Product/1
  Ki.dT+ Ipv,n/1 -> Product/2
  Product/1 -> Ipv/1
  Subsystem2/1(dT) -> Ki.dT/2
  T/1 -> Subsystem2/1(T)

== system GMPP2/PV5/Subsystem1 ==
  T(°C) : Inport
  Constant1 : Constant  Value=273.15
  V+Rs.I1 : Sum
  T(K) : Outport
  wires:
  Constant1/1 -> V+Rs.I1/2
  T(°C)/1 -> V+Rs.I1/1
  V+Rs.I1/1 -> T(K)/1

== system GMPP2/PV5/Subsystem3 ==
  T : Inport
  Divide : Product  Inputs=**/
  K : Constant  Value=1.38e-23
  q : Constant  Value=1.6e-19
  Vt : Outport
  wires:
  K/1 -> Divide/1
  T/1 -> Divide/2
  q/1 -> Divide/3
  Divide/1 -> Vt/1

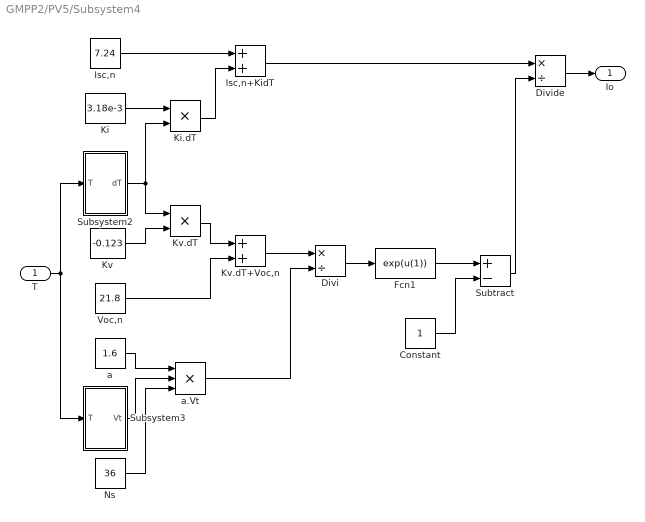
== system GMPP2/PV5/Subsystem4 ==
  T : Inport
  Constant : Constant
  Divi : Product  Inputs=*/
  Divide : Product  Inputs=*/
  Fcn1 : Fcn  Expr=exp(u(1))
  Isc,n : Constant  Value=7.24
  Isc,n+KidT : Sum
  Ki : Constant  Value=3.18e-3
  Ki.dT : Product  RndMeth=Zero
  Kv : Constant  Value=-0.123
  Kv.dT : Product  RndMeth=Zero
  Kv.dT+Voc,n : Sum
  Ns : Constant  Value=36
  Subsystem2 : Subsystem
  Subsystem3 : Subsystem
  Subtract : Sum  Inputs=+-
  Voc,n : Constant  Value=21.8
  a : Constant  Value=1.6
  a.Vt : Product  Inputs=3  RndMeth=Zero
  Io : Outport
  wires:
  Subsystem2/1(dT) -> Kv.dT/1, Ki.dT/2
  Kv/1 -> Kv.dT/2
  Kv.dT/1 -> Kv.dT+Voc,n/1
  Voc,n/1 -> Kv.dT+Voc,n/2
  a/1 -> a.Vt/1
  Subsystem3/1(Vt) -> a.Vt/2
  Kv.dT+Voc,n/1 -> Divi/1
  a.Vt/1 -> Divi/2
  Divi/1 -> Fcn1/1
  Fcn1/1 -> Subtract/1
  Constant/1 -> Subtract/2
  Ki/1 -> Ki.dT/1
  Isc,n/1 -> Isc,n+KidT/1
  Ki.dT/1 -> Isc,n+KidT/2
  Isc,n+KidT/1 -> Divide/1
  Subtract/1 -> Divide/2
  Divide/1 -> Io/1
  T/1 -> Subsystem2/1(T), Subsystem3/1(T)
  Ns/1 -> a.Vt/3

== system GMPP2/PV7/Subsystem ==
  G : Inport
  T : Inport  Port=2
  G/Gn : Product  Inputs=*/
  Gn : Constant  Value=1000
  Ipv,n : Constant  Value=7.24
  Ki : Constant  Value=3.18e-3
  Ki.dT : Product  RndMeth=Zero
  Ki.dT+ Ipv,n : Sum
  Product : Product  RndMeth=Zero
  Subsystem2 : Subsystem
  Ipv : Outport
  wires:
  Ki/1 -> Ki.dT/1
  Ipv,n/1 -> Ki.dT+ Ipv,n/1
  Ki.dT/1 -> Ki.dT+ Ipv,n/2
  G/1 -> G/Gn/1
  Gn/1 -> G/Gn/2
  G/Gn/1 -> Product/1
  Ki.dT+ Ipv,n/1 -> Product/2
  Product/1 -> Ipv/1
  Subsystem2/1(dT) -> Ki.dT/2
  T/1 -> Subsystem2/1(T)

== system GMPP2/PV7/Subsystem1 ==
  T(°C) : Inport
  Constant1 : Constant  Value=273.15
  V+Rs.I1 : Sum
  T(K) : Outport
  wires:
  Constant1/1 -> V+Rs.I1/2
  T(°C)/1 -> V+Rs.I1/1
  V+Rs.I1/1 -> T(K)/1

== system GMPP2/PV7/Subsystem3 ==
  T : Inport
  Divide : Product  Inputs=**/
  K : Constant  Value=1.38e-23
  q : Constant  Value=1.6e-19
  Vt : Outport
  wires:
  K/1 -> Divide/1
  T/1 -> Divide/2
  q/1 -> Divide/3
  Divide/1 -> Vt/1

== system GMPP2/PV7/Subsystem4 ==
  T : Inport
  Constant : Constant
  Divi : Product  Inputs=*/
  Divide : Product  Inputs=*/
  Fcn1 : Fcn  Expr=exp(u(1))
  Isc,n : Constant  Value=7.24
  Isc,n+KidT : Sum
  Ki : Constant  Value=3.18e-3
  Ki.dT : Product  RndMeth=Zero
  Kv : Constant  Value=-0.123
  Kv.dT : Product  RndMeth=Zero
  Kv.dT+Voc,n : Sum
  Ns : Constant  Value=36
  Subsystem2 : Subsystem
  Subsystem3 : Subsystem
  Subtract : Sum  Inputs=+-
  Voc,n : Constant  Value=21.8
  a : Constant  Value=1.6
  a.Vt : Product  Inputs=3  RndMeth=Zero
  Io : Outport
  wires:
  Subsystem2/1(dT) -> Kv.dT/1, Ki.dT/2
  Kv/1 -> Kv.dT/2
  Kv.dT/1 -> Kv.dT+Voc,n/1
  Voc,n/1 -> Kv.dT+Voc,n/2
  a/1 -> a.Vt/1
  Subsystem3/1(Vt) -> a.Vt/2
  Kv.dT+Voc,n/1 -> Divi/1
  a.Vt/1 -> Divi/2
  Divi/1 -> Fcn1/1
  Fcn1/1 -> Subtract/1
  Constant/1 -> Subtract/2
  Ki/1 -> Ki.dT/1
  Isc,n/1 -> Isc,n+KidT/1
  Ki.dT/1 -> Isc,n+KidT/2
  Isc,n+KidT/1 -> Divide/1
  Subtract/1 -> Divide/2
  Divide/1 -> Io/1
  T/1 -> Subsystem2/1(T), Subsystem3/1(T)
  Ns/1 -> a.Vt/3

== system GMPP2/pwm/saw wave ==
  Integrator : Integrator  ExternalReset=rising  ShowStatePort=on
  Sign : Signum
  Sum : Sum  Inputs=+-|
  fs : Constant  Value=fs
  one : Constant
  Out1 : Outport
  wires:
  Integrator/1 -> Out1/1
  Sum/1 -> Sign/1
  fs/1 -> Integrator/1
  one/1 -> Sum/2
  Sign/1 -> Integrator/2
  Integrator/State -> Sum/1

== system GMPP2/ANN/Layer 1/Delays 1 ==
  "p{1}" : Inport  PortDimensions=2
      mask Display: e = 0.06;c1 = [120 230 180]/255;c2 = ([120 230 180]+0)/(256+128);c3 = ([120 230 180]+128)/(256+128);patch([0 1 1 0],[0 0 1 1],c1);patch([0 1 1 1-e 1-e 0+e],[0 0 1 1-e 0+e 0+e],c2);patch([0 0 1 1-e 0+e 0+e],[0 1 1 1-e 1-e 0+e],c3);plot([0 1 1 0 0],[0 0 1 1 0]);
  mux : Mux  Inputs=1
      mask Display: e = 0.06;c1 = [120 150 230]/255;c2 = ([120 150 230]+0)/383;c3 = ([120 150 230]+128)/383;patch([0 1 1 0],[0 0 1 1],c1);patch([0 1 1 1-e 1-e 0+e],[0 0 1 1-e 0+e 0+e],c2);patch([0 0 1 1-e 0+e 0+e],[0 1 1 1-e 1-e 0+e],c3);plot([0 1 1 0 0],[0 0 1 1 0]);disp('Mux')
  "pd{1,1}" : Outport
      mask Display: e = 0.06;c1 = [120 230 180]/255;c2 = ([120 230 180]+0)/(256+128);c3 = ([120 230 180]+128)/(256+128);patch([0 1 1 0],[0 0 1 1],c1);patch([0 1 1 1-e 1-e 0+e],[0 0 1 1-e 0+e 0+e],c2);patch([0 0 1 1-e 0+e 0+e],[0 1 1 1-e 1-e 0+e],c3);plot([0 1 1 0 0],[0 0 1 1 0]);
  wires:
  "p{1}"/1 -> mux/1
  mux/1 -> "pd{1,1}"/1

== system GMPP2/ANN/Layer 1/IW{1,1} ==
  "pd{1,1}" : Inport  PortDimensions=2
      mask Display: e = 0.06;c1 = [120 230 180]/255;c2 = ([120 230 180]+0)/(256+128);c3 = ([120 230 180]+128)/(256+128);patch([0 1 1 0],[0 0 1 1],c1);patch([0 1 1 1-e 1-e 0+e],[0 0 1 1-e 0+e 0+e],c2);patch([0 0 1 1-e 0+e 0+e],[0 1 1 1-e 1-e 0+e],c3);plot([0 1 1 0 0],[0 0 1 1 0]);
  "IW{1,1}(1,:)'" : Constant  Value=[0.61591302444223783;-0.060606567497894726]
      mask Display: e = 0.06;c1 = [120 150 230]/255;c2 = ([120 150 230]+0)/383;c3 = ([120 150 230]+128)/383;patch([0 1 1 0],[0 0 1 1],c1);patch([0 1 1 1-e 1-e 0+e],[0 0 1 1-e 0+e 0+e],c2);patch([0 0 1 1-e 0+e 0+e],[0 1 1 1-e 1-e 0+e],c3);plot([0 1 1 0 0],[0 0 1 1 0]);disp('Weights');
  Mux : Mux  Inputs=1
      mask Display: e = 0.06;c1 = [120 150 230]/255;c2 = ([120 150 230]+0)/383;c3 = ([120 150 230]+128)/383;patch([0 1 1 0],[0 0 1 1],c1);patch([0 1 1 1-e 1-e 0+e],[0 0 1 1-e 0+e 0+e],c2);patch([0 0 1 1-e 0+e 0+e],[0 1 1 1-e 1-e 0+e],c3);plot([0 1 1 0 0],[0 0 1 1 0]);disp('Mux');
  dotprod1 : neural/Weight Functions/dotprod
  "iz{1,1}" : Outport
      mask Display: e = 0.06;c1 = [120 230 180]/255;c2 = ([120 230 180]+0)/(256+128);c3 = ([120 230 180]+128)/(256+128);patch([0 1 1 0],[0 0 1 1],c1);patch([0 1 1 1-e 1-e 0+e],[0 0 1 1-e 0+e 0+e],c2);patch([0 0 1 1-e 0+e 0+e],[0 1 1 1-e 1-e 0+e],c3);plot([0 1 1 0 0],[0 0 1 1 0]);
  wires:
  "IW{1,1}(1,:)'"/1 -> dotprod1/1
  "pd{1,1}"/1 -> dotprod1/2
  dotprod1/1 -> Mux/1
  Mux/1 -> "iz{1,1}"/1

== system GMPP2/ANN/Layer 2/Delays 1 ==
  "p{2}" : Inport  PortDimensions=1
      mask Display: e = 0.06;c1 = [120 230 180]/255;c2 = ([120 230 180]+0)/(256+128);c3 = ([120 230 180]+128)/(256+128);patch([0 1 1 0],[0 0 1 1],c1);patch([0 1 1 1-e 1-e 0+e],[0 0 1 1-e 0+e 0+e],c2);patch([0 0 1 1-e 0+e 0+e],[0 1 1 1-e 1-e 0+e],c3);plot([0 1 1 0 0],[0 0 1 1 0]);
  mux : Mux  Inputs=1
      mask Display: e = 0.06;c1 = [120 150 230]/255;c2 = ([120 150 230]+0)/383;c3 = ([120 150 230]+128)/383;patch([0 1 1 0],[0 0 1 1],c1);patch([0 1 1 1-e 1-e 0+e],[0 0 1 1-e 0+e 0+e],c2);patch([0 0 1 1-e 0+e 0+e],[0 1 1 1-e 1-e 0+e],c3);plot([0 1 1 0 0],[0 0 1 1 0]);disp('Mux')
  "pd{2,1}" : Outport
      mask Display: e = 0.06;c1 = [120 230 180]/255;c2 = ([120 230 180]+0)/(256+128);c3 = ([120 230 180]+128)/(256+128);patch([0 1 1 0],[0 0 1 1],c1);patch([0 1 1 1-e 1-e 0+e],[0 0 1 1-e 0+e 0+e],c2);patch([0 0 1 1-e 0+e 0+e],[0 1 1 1-e 1-e 0+e],c3);plot([0 1 1 0 0],[0 0 1 1 0]);
  wires:
  "p{2}"/1 -> mux/1
  mux/1 -> "pd{2,1}"/1

== system GMPP2/ANN/Layer 2/LW{2,1} ==
  "ad{2,1}" : Inport  PortDimensions=1
      mask Display: e = 0.06;c1 = [120 230 180]/255;c2 = ([120 230 180]+0)/(256+128);c3 = ([120 230 180]+128)/(256+128);patch([0 1 1 0],[0 0 1 1],c1);patch([0 1 1 1-e 1-e 0+e],[0 0 1 1-e 0+e 0+e],c2);patch([0 0 1 1-e 0+e 0+e],[0 1 1 1-e 1-e 0+e],c3);plot([0 1 1 0 0],[0 0 1 1 0]);
  "IW{2,1}(1,:)'" : Constant  Value=24.89320145293242
      mask Display: e = 0.06;c1 = [120 150 230]/255;c2 = ([120 150 230]+0)/383;c3 = ([120 150 230]+128)/383;patch([0 1 1 0],[0 0 1 1],c1);patch([0 1 1 1-e 1-e 0+e],[0 0 1 1-e 0+e 0+e],c2);patch([0 0 1 1-e 0+e 0+e],[0 1 1 1-e 1-e 0+e],c3);plot([0 1 1 0 0],[0 0 1 1 0]);disp('weights');
  Mux : Mux  Inputs=1
      mask Display: e = 0.06;c1 = [120 150 230]/255;c2 = ([120 150 230]+0)/383;c3 = ([120 150 230]+128)/383;patch([0 1 1 0],[0 0 1 1],c1);patch([0 1 1 1-e 1-e 0+e],[0 0 1 1-e 0+e 0+e],c2);patch([0 0 1 1-e 0+e 0+e],[0 1 1 1-e 1-e 0+e],c3);plot([0 1 1 0 0],[0 0 1 1 0]);disp('Mux');
  dotprod1 : neural/Weight Functions/dotprod
  "lz{2,1}" : Outport
      mask Display: e = 0.06;c1 = [120 230 180]/255;c2 = ([120 230 180]+0)/(256+128);c3 = ([120 230 180]+128)/(256+128);patch([0 1 1 0],[0 0 1 1],c1);patch([0 1 1 1-e 1-e 0+e],[0 0 1 1-e 0+e 0+e],c2);patch([0 0 1 1-e 0+e 0+e],[0 1 1 1-e 1-e 0+e],c3);plot([0 1 1 0 0],[0 0 1 1 0]);
  wires:
  "IW{2,1}(1,:)'"/1 -> dotprod1/1
  "ad{2,1}"/1 -> dotprod1/2
  dotprod1/1 -> Mux/1
  Mux/1 -> "lz{2,1}"/1

== system GMPP2/PV1/Subsystem/Subsystem2 ==
  T : Inport
  Subtrac : Sum  Inputs=+-
  Tn : Constant  Value=298.15
  dT : Outport
  wires:
  T/1 -> Subtrac/1
  Tn/1 -> Subtrac/2
  Subtrac/1 -> dT/1

== system GMPP2/PV1/Subsystem4/Subsystem2 ==
  T : Inport
  Subtrac : Sum  Inputs=+-
  Tn : Constant  Value=298.15
  dT : Outport
  wires:
  T/1 -> Subtrac/1
  Tn/1 -> Subtrac/2
  Subtrac/1 -> dT/1

== system GMPP2/PV1/Subsystem4/Subsystem3 ==
  T : Inport
  Divide : Product  Inputs=**/
  K : Constant  Value=1.38e-23
  q : Constant  Value=1.6e-19
  Vt : Outport
  wires:
  K/1 -> Divide/1
  T/1 -> Divide/2
  q/1 -> Divide/3
  Divide/1 -> Vt/1

== system GMPP2/PV2/Subsystem/Subsystem2 ==
  T : Inport
  Subtrac : Sum  Inputs=+-
  Tn : Constant  Value=298.15
  dT : Outport
  wires:
  T/1 -> Subtrac/1
  Tn/1 -> Subtrac/2
  Subtrac/1 -> dT/1

== system GMPP2/PV2/Subsystem4/Subsystem2 ==
  T : Inport
  Subtrac : Sum  Inputs=+-
  Tn : Constant  Value=298.15
  dT : Outport
  wires:
  T/1 -> Subtrac/1
  Tn/1 -> Subtrac/2
  Subtrac/1 -> dT/1

== system GMPP2/PV2/Subsystem4/Subsystem3 ==
  T : Inport
  Divide : Product  Inputs=**/
  K : Constant  Value=1.38e-23
  q : Constant  Value=1.6e-19
  Vt : Outport
  wires:
  K/1 -> Divide/1
  T/1 -> Divide/2
  q/1 -> Divide/3
  Divide/1 -> Vt/1

== system GMPP2/PV3/Subsystem/Subsystem2 ==
  T : Inport
  Subtrac : Sum  Inputs=+-
  Tn : Constant  Value=298.15
  dT : Outport
  wires:
  T/1 -> Subtrac/1
  Tn/1 -> Subtrac/2
  Subtrac/1 -> dT/1

== system GMPP2/PV3/Subsystem4/Subsystem2 ==
  T : Inport
  Subtrac : Sum  Inputs=+-
  Tn : Constant  Value=298.15
  dT : Outport
  wires:
  T/1 -> Subtrac/1
  Tn/1 -> Subtrac/2
  Subtrac/1 -> dT/1

== system GMPP2/PV3/Subsystem4/Subsystem3 ==
  T : Inport
  Divide : Product  Inputs=**/
  K : Constant  Value=1.38e-23
  q : Constant  Value=1.6e-19
  Vt : Outport
  wires:
  K/1 -> Divide/1
  T/1 -> Divide/2
  q/1 -> Divide/3
  Divide/1 -> Vt/1

== system GMPP2/PV4/Subsystem/Subsystem2 ==
  T : Inport
  Subtrac : Sum  Inputs=+-
  Tn : Constant  Value=298.15
  dT : Outport
  wires:
  T/1 -> Subtrac/1
  Tn/1 -> Subtrac/2
  Subtrac/1 -> dT/1

== system GMPP2/PV4/Subsystem4/Subsystem2 ==
  T : Inport
  Subtrac : Sum  Inputs=+-
  Tn : Constant  Value=298.15
  dT : Outport
  wires:
  T/1 -> Subtrac/1
  Tn/1 -> Subtrac/2
  Subtrac/1 -> dT/1

== system GMPP2/PV4/Subsystem4/Subsystem3 ==
  T : Inport
  Divide : Product  Inputs=**/
  K : Constant  Value=1.38e-23
  q : Constant  Value=1.6e-19
  Vt : Outport
  wires:
  K/1 -> Divide/1
  T/1 -> Divide/2
  q/1 -> Divide/3
  Divide/1 -> Vt/1

== system GMPP2/PV5/Subsystem/Subsystem2 ==
  T : Inport
  Subtrac : Sum  Inputs=+-
  Tn : Constant  Value=298.15
  dT : Outport
  wires:
  T/1 -> Subtrac/1
  Tn/1 -> Subtrac/2
  Subtrac/1 -> dT/1

== system GMPP2/PV5/Subsystem4/Subsystem2 ==
  T : Inport
  Subtrac : Sum  Inputs=+-
  Tn : Constant  Value=298.15
  dT : Outport
  wires:
  T/1 -> Subtrac/1
  Tn/1 -> Subtrac/2
  Subtrac/1 -> dT/1
